simulink subsystem "estimator_subsystem"  (R2024b)
settings: Solver=VariableStepAuto  StartTime=0.0  StopTime=10.0  RelTol=1e-3
settings Model: Creator=finnb  LastModifiedBy=finnb

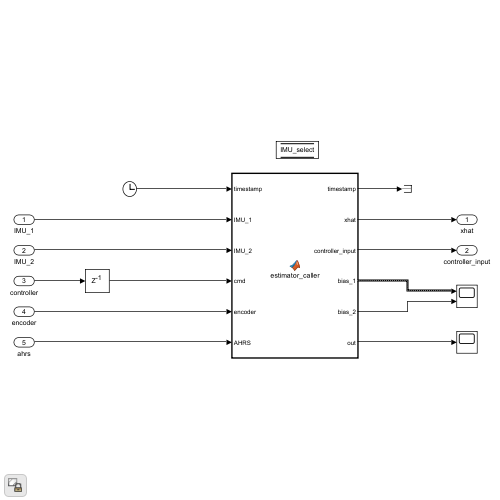
[thumbnail: Simulink's stored preview of the top-level diagram]
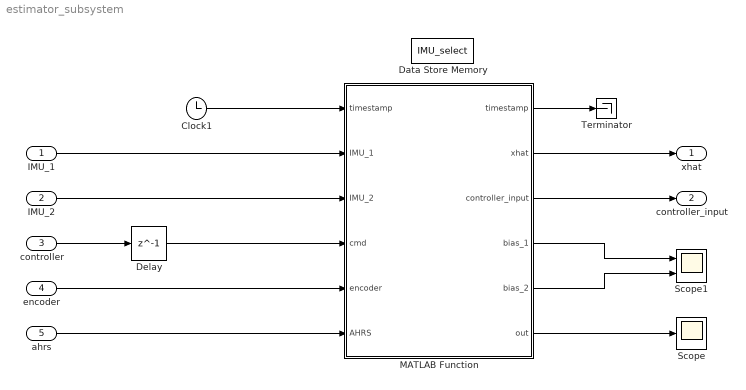
== system estimator_subsystem ==
  IMU_1 : Inport
  IMU_2 : Inport  Port=2
  controller : Inport  Port=3
  encoder : Inport  Port=4
  ahrs : Inport  Port=5
  Clock1 : Clock
  Data Store Memory : DataStoreMemory  DataStoreName=IMU_select  WriteAfterWriteMsg=warning  InitialValue=[0 0]  ShowAdditionalParam=off  OutDataTypeStr=double
  Delay : Delay  DelayLength=1
  MATLAB Function : MATLAB Function  TreatAsAtomicUnit=on
  Scope : Scope
  Scope1 : Scope  NumInputPorts=2
  Terminator : Terminator
  xhat : Outport
  controller_input : Outport  Port=2
  wires:
  IMU_1/1 -> MATLAB Function/2(IMU_1)
  Clock1/1 -> MATLAB Function/1("timestamp ")
  IMU_2/1 -> MATLAB Function/3(IMU_2)
  MATLAB Function/2(xhat) -> xhat/1
  Delay/1 -> MATLAB Function/4(cmd)
  encoder/1 -> MATLAB Function/5(encoder)
  controller/1 -> Delay/1
  MATLAB Function/1(timestamp) -> Terminator/1
  MATLAB Function/3(controller_input) -> controller_input/1
  MATLAB Function/6(out) -> Scope/1
  MATLAB Function/4(bias_1) -> Scope1/1
  MATLAB Function/5(bias_2) -> Scope1/2
  ahrs/1 -> MATLAB Function/6(AHRS)

== matlab function estimator_subsystem/MATLAB Function ==
  settings: updateMethod=DISCRETE  sampleTime=samplingrate
  data: timestamp output; timestamp input; IMU_1 input; IMU_2 input; cmd input; xhat output size=13; controller_input output; bias_1 output size=[10, 3]; bias_2 output; encoder input; IMU_select data_store_memory; out output; AHRS input
function [timestamp, xhat, controller_input, bias_1, bias_2, out] = estimator_caller(timestamp, IMU_1, IMU_2, cmd, encoder, AHRS)

    global IMU_select 
    % IMU_select = [1, 0];

    [IMU_1, IMU_2] = imu_handler(IMU_1, IMU_2, IMU_select);

    [xhat, Phat, controller_input, bias_1, bias_2] = estimator_module(timestamp, IMU_1, IMU_2, cmd, encoder, AHRS);

    out = [norm(Phat, 1), norm(Phat, 2), norm(Phat, Inf)];
end
